simulink model "UberSpurs"  (R2015b)
settings: Solver=VariableStepAuto  StartTime=0.0  StopTime=5000  RelTol=1e-3
libraries: simulink x54
(part 1 of 6)
settings Model: Creator=tsprock3  LastModifiedBy=tsprock3
settings DebuggingCC: UnconnectedOutputMsg=error

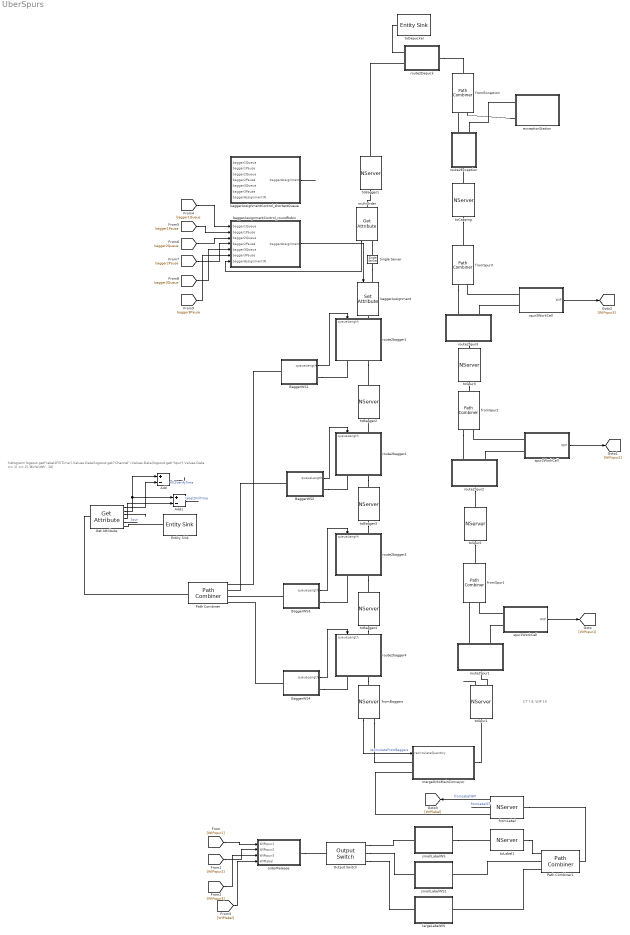
== system UberSpurs ==
  note: histogram(logsout.get('label2FillTime').Values.Data(logsout.get('Channel').Values.Data(logsout.get('Spur').Values.Data == 1) == 2),'BinWidth', 10)
  note: CT 7.8, WIP 19
  Add : Sum  Inputs=+-
  Add1 : Sum  Inputs=+-
  BaggerWS1 : Subsystem
  BaggerWS2 : Subsystem
  BaggerWS3 : Subsystem
  BaggerWS4 : Subsystem
  Entity Sink : EntitySink
  Get Attribute : GetAttribute  AttributeName=FillTime|VerifyTime|Channel|LabelTime|Spur  AttributeMissing=Error|Error|Error|Error|Error  AttributeDefaultValue=1|1|1|1|1  AttributeTreatAsVector=1|1|1|1|1  AttributeSendTiming=After entity departure|After entity departure|After entity departure|After entity departure|After entity departure  EvaluatedDefaultAttributeValue={ [];[];[];[];[]}
      settings: OutputPortMap=o1,o2,o3,o4,o5
  Output Switch : OutputSwitch  SwitchingCriterion=From attribute  AttributeName=Labeler  InitialConditionsOpt=on
  Path Combiner : PathCombiner  NumberInputPorts=4
  Path Combiner1 : PathCombiner
  Single Server : SingleServer  ServiceTime=0
  baggerAssignment : SetAttribute  AttributeName=Bagger  AttributeFrom=Signal port  EvaluatedAttributeValue={ []}
  baggerAssignmentControl_roundRobin : Stateflow chart  TreatAsAtomicUnit=on
  baggerAssignmentControl_shortestQueue : Stateflow chart  TreatAsAtomicUnit=on
  exceptionStation : Subsystem
  fromBaggers : NServer  NumberOfServers=12  ServiceTime=4.9  StatNumberInBlock=on
      settings: OutputPortMap=o1
  fromException : PathCombiner  NumberInputPorts=2
  fromLabel : NServer  NumberOfServers=45  ServiceTime=37  StatNumberInBlock=on  StatAverageWait=on
      settings: OutputPortMap=o1,o4
  fromSpur1 : PathCombiner  NumberInputPorts=2  InputPortPrecedence=Round robin
  fromSpur2 : PathCombiner  NumberInputPorts=2  InputPortPrecedence=Round robin
  fromSpur3 : PathCombiner  NumberInputPorts=2  InputPortPrecedence=Round robin
  largeLabelWS : Subsystem
  mergeOntoMainConveyor : Subsystem
  multiOrder : GetAttribute  AttributeName=Bagger  EvaluatedDefaultAttributeValue={ []}
      settings: OutputPortMap=o1
  orderRelease : Subsystem
  route2Depuck : Subsystem
  route2Exception : Subsystem
  route2Spur1 : Subsystem
  route2Spur2 : Subsystem
  route2Spur3 : Subsystem
  route2bagger1 : Subsystem
  route2bagger2 : Subsystem
  route2bagger3 : Subsystem
  route2bagger4 : Subsystem
  smallLabelWS : Subsystem
  smallLabelWS1 : Subsystem
  spur1WorkCell : Subsystem
  spur2WorkCell : Subsystem
  spur3WorkCell : Subsystem
  toBagger{1..4} (4 alike) : NServer  NumberOfServers=30  ServiceTime=12.1
  toCapping : NServer  NumberOfServers=25  ServiceTime=10.4
  toDepucker : EntitySink
  toLabel1 : NServer  NumberOfServers=22  ServiceTime=8
  toSpur1 : NServer  NumberOfServers=19  ServiceTime=7.79  StatNumberInBlock=on
      settings: OutputPortMap=o1
  toSpur2 : NServer  NumberOfServers=20  ServiceTime=8.3
  toSpur3 : NServer  NumberOfServers=20  ServiceTime=8.3
  wires:
  Add/1 -> ?  "fill2VerifyTime"
  Get Attribute/3 -> ?
  Get Attribute/2 -> Add1/1, Add/1
  Get Attribute/1 -> Add/2
  Add1/1 -> ?  "label2FillTime"
  Get Attribute/4 -> Add1/2
  spur1WorkCell/1(WIP) -> [WIPspur1]
  [WIPspur1] -> orderRelease/1(WIPspur1)
  BaggerWS4/1(queueLength) -> route2bagger4/1(queueLength)
  BaggerWS3/1(queueLength) -> route2bagger3/1(queueLength)
  BaggerWS2/1(queueLength) -> route2bagger2/1(queueLength)
  BaggerWS1/1(queueLength) -> route2bagger1/1(queueLength)
  spur2WorkCell/1(WIP) -> [WIPspur2]
  [WIPspur2] -> orderRelease/2(WIPspur2)
  fromLabel/2 -> ?  "fromLabelCT"
  fromLabel/1 -> [WIPlabel]  "fromLabelWIP"
  [WIPspur3] -> orderRelease/3(WIPspur3)
  [WIPlabel] -> orderRelease/4(WIPlabel)
  toSpur1/1 -> ?
  Get Attribute/5 -> ?  "Spur"
  spur3WorkCell/1(WIP) -> [WIPspur3]
  fromBaggers/1 -> mergeOntoMainConveyor/1(recirculateQuantity)  "recirculateFromBaggers"
  baggerAssignmentControl_roundRobin/1(baggerAssignment) -> baggerAssignment/1
  multiOrder/1 -> baggerAssignmentControl_roundRobin/7(baggerAssignmentIN)
  [bagger1Queue] -> baggerAssignmentControl_roundRobin/1(bagger1Queue)
  [bagger1Pause] -> baggerAssignmentControl_roundRobin/2(bagger1Pause)
  [bagger2Queue] -> baggerAssignmentControl_roundRobin/3(bagger2Queue)
  [bagger2Pause] -> baggerAssignmentControl_roundRobin/4(bagger2Pause)
  [bagger3Queue] -> baggerAssignmentControl_roundRobin/5(bagger3Queue)
  [bagger3Pause] -> baggerAssignmentControl_roundRobin/6(bagger3Pause)
  baggerAssignmentControl_shortestQueue/1(baggerAssignment) -> ?
  connections:
  Get Attribute/RConn1 -- Entity Sink/LConn1
  spur1WorkCell/LConn1 -- fromSpur1/LConn2
  toSpur1/RConn1 -- route2Spur1/LConn1
  route2Spur1/RConn2 -- spur1WorkCell/LConn2
  route2Spur1/RConn1 -- fromSpur1/LConn1
  BaggerWS1/LConn1 -- Path Combiner/LConn1
  BaggerWS3/LConn1 -- Path Combiner/LConn3
  Path Combiner/RConn1 -- Get Attribute/LConn1
  Output Switch/RConn2 -- smallLabelWS1/LConn1
  toLabel1/RConn1 -- Path Combiner1/LConn1
  BaggerWS4/RConn1 -- route2bagger4/RConn1
  route2bagger4/RConn2 -- fromBaggers/LConn1
  toBagger4/RConn1 -- route2bagger4/LConn1
  orderRelease/RConn1 -- Output Switch/LConn1
  BaggerWS3/RConn1 -- route2bagger3/RConn1
  route2bagger3/RConn2 -- toBagger4/LConn1
  BaggerWS2/LConn1 -- Path Combiner/LConn2
  toBagger3/RConn1 -- route2bagger3/LConn1
  route2bagger2/RConn2 -- toBagger3/LConn1
  BaggerWS2/RConn1 -- route2bagger2/RConn1
  toBagger2/RConn1 -- route2bagger2/LConn1
  route2bagger1/RConn2 -- toBagger2/LConn1
  BaggerWS1/RConn1 -- route2bagger1/RConn1
  toSpur2/LConn1 -- fromSpur1/RConn1
  Path Combiner1/LConn2 -- smallLabelWS1/RConn1
  fromLabel/LConn1 -- Path Combiner1/RConn1
  BaggerWS4/LConn1 -- Path Combiner/LConn4
  spur2WorkCell/LConn2 -- route2Spur2/RConn2
  route2Spur2/LConn1 -- toSpur2/RConn1
  fromSpur2/LConn1 -- route2Spur2/RConn1
  toSpur3/LConn1 -- fromSpur2/RConn1
  spur2WorkCell/LConn1 -- fromSpur2/LConn2
  spur3WorkCell/LConn1 -- fromSpur3/LConn2
  fromSpur3/LConn1 -- route2Spur3/RConn1
  spur3WorkCell/LConn2 -- route2Spur3/RConn2
  route2Spur3/LConn1 -- toSpur3/RConn1
  toCapping/LConn1 -- fromSpur3/RConn1
  toCapping/RConn1 -- route2Exception/LConn1
  route2Exception/RConn1 -- fromException/LConn1
  route2Exception/RConn2 -- exceptionStation/LConn1
  exceptionStation/LConn2 -- fromException/LConn2
  route2Depuck/LConn1 -- fromException/RConn1
  route2Depuck/RConn2 -- toBagger1/LConn1
  toDepucker/LConn1 -- route2Depuck/RConn1
  Path Combiner1/LConn3 -- largeLabelWS/RConn1
  Output Switch/RConn3 -- largeLabelWS/LConn1
  smallLabelWS/RConn1 -- toLabel1/LConn1
  Output Switch/RConn1 -- smallLabelWS/LConn1
  fromBaggers/RConn1 -- mergeOntoMainConveyor/LConn1
  mergeOntoMainConveyor/RConn1 -- toSpur1/LConn1
  fromLabel/RConn1 -- mergeOntoMainConveyor/LConn2
  baggerAssignment/RConn1 -- route2bagger1/LConn1
  multiOrder/LConn1 -- toBagger1/RConn1
  Single Server/RConn1 -- baggerAssignment/LConn1
  Single Server/LConn1 -- multiOrder/RConn1

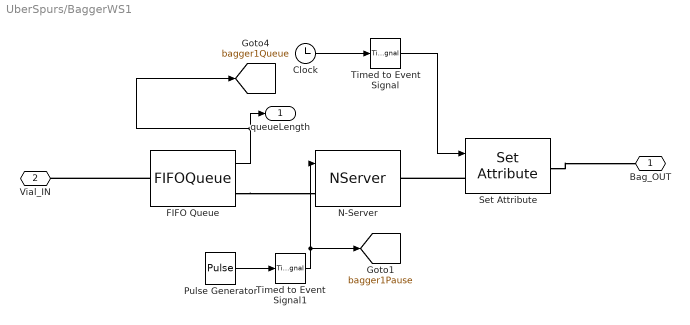
== system UberSpurs/BaggerWS1 ==
  Clock : Clock
  FIFO Queue : FIFOQueue  Capacity=26  StatNumberInBlock=on
      settings: OutputPortMap=o1
  N-Server : NServer  NumberOfServers=1  ServiceTime=6  AllowServiceControl=on
      settings: InputPortMap=u1
  Pulse Generator : DiscretePulseGenerator  PulseType=Time based  Period=100  PulseWidth=10
  Set Attribute : SetAttribute  AttributeName=BagTime  AttributeFrom=Signal port  EvaluatedAttributeValue={ []}
  Timed to Event Signal : TimedToEventSignal
  Timed to Event Signal1 : TimedToEventSignal
  Bag_OUT : PMIOPort  Port=1  Side=Left
  Vial_IN : PMIOPort  Port=2  Side=Right
  queueLength : Outport
  tag scope: bagger1Pause=global, bagger1Queue=global
  wires:
  Clock/1 -> Timed to Event Signal/1
  Timed to Event Signal/1 -> Set Attribute/1
  FIFO Queue/1 -> [bagger1Queue], queueLength/1
  Pulse Generator/1 -> Timed to Event Signal1/1
  Timed to Event Signal1/1 -> [bagger1Pause], N-Server/1
  connections:
  FIFO Queue/LConn1 -- Vial_IN/RConn1
  FIFO Queue/RConn1 -- N-Server/LConn1
  Set Attribute/LConn1 -- N-Server/RConn1
  Set Attribute/RConn1 -- Bag_OUT/RConn1

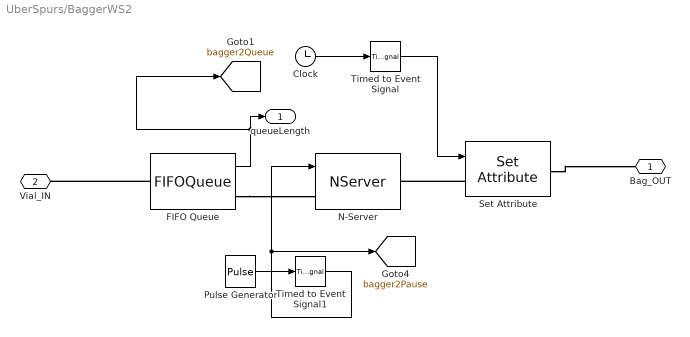
== system UberSpurs/BaggerWS2 ==
  Clock : Clock
  FIFO Queue : FIFOQueue  Capacity=26  StatNumberInBlock=on
      settings: OutputPortMap=o1
  N-Server : NServer  NumberOfServers=1  ServiceTime=6  AllowServiceControl=on
      settings: InputPortMap=u1
  Pulse Generator : DiscretePulseGenerator  PulseType=Time based  Period=100  PulseWidth=10  PhaseDelay=250
  Set Attribute : SetAttribute  AttributeName=BagTime  AttributeFrom=Signal port  EvaluatedAttributeValue={ []}
  Timed to Event Signal : TimedToEventSignal
  Timed to Event Signal1 : TimedToEventSignal
  Bag_OUT : PMIOPort  Port=1  Side=Left
  Vial_IN : PMIOPort  Port=2  Side=Right
  queueLength : Outport
  tag scope: bagger2Pause=global, bagger2Queue=global
  wires:
  Clock/1 -> Timed to Event Signal/1
  Timed to Event Signal/1 -> Set Attribute/1
  FIFO Queue/1 -> [bagger2Queue], queueLength/1
  Pulse Generator/1 -> Timed to Event Signal1/1
  Timed to Event Signal1/1 -> [bagger2Pause], N-Server/1
  connections:
  FIFO Queue/LConn1 -- Vial_IN/RConn1
  FIFO Queue/RConn1 -- N-Server/LConn1
  Set Attribute/LConn1 -- N-Server/RConn1
  Set Attribute/RConn1 -- Bag_OUT/RConn1

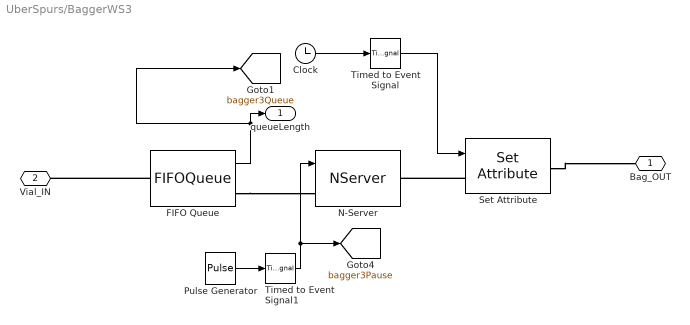
== system UberSpurs/BaggerWS3 ==
  Clock : Clock
  FIFO Queue : FIFOQueue  Capacity=26  StatNumberInBlock=on
      settings: OutputPortMap=o1
  N-Server : NServer  NumberOfServers=1  ServiceTime=6  AllowServiceControl=on
      settings: InputPortMap=u1
  Pulse Generator : DiscretePulseGenerator  PulseType=Time based  Period=100  PulseWidth=10  PhaseDelay=500
  Set Attribute : SetAttribute  AttributeName=BagTime  AttributeFrom=Signal port  EvaluatedAttributeValue={ []}
  Timed to Event Signal : TimedToEventSignal
  Timed to Event Signal1 : TimedToEventSignal
  Bag_OUT : PMIOPort  Port=1  Side=Left
  Vial_IN : PMIOPort  Port=2  Side=Right
  queueLength : Outport
  tag scope: bagger3Pause=global, bagger3Queue=global
  wires:
  Clock/1 -> Timed to Event Signal/1
  Timed to Event Signal/1 -> Set Attribute/1
  FIFO Queue/1 -> [bagger3Queue], queueLength/1
  Pulse Generator/1 -> Timed to Event Signal1/1
  Timed to Event Signal1/1 -> [bagger3Pause], N-Server/1
  connections:
  FIFO Queue/LConn1 -- Vial_IN/RConn1
  FIFO Queue/RConn1 -- N-Server/LConn1
  Set Attribute/LConn1 -- N-Server/RConn1
  Set Attribute/RConn1 -- Bag_OUT/RConn1

== system UberSpurs/BaggerWS4 ==
  Clock : Clock
  FIFO Queue : FIFOQueue  Capacity=26  StatNumberInBlock=on
      settings: OutputPortMap=o1
  N-Server : NServer  NumberOfServers=1  ServiceTime=6  AllowServiceControl=on
      settings: InputPortMap=u1
  Pulse Generator : DiscretePulseGenerator  PulseType=Time based  Period=100  PulseWidth=10  PhaseDelay=750
  Set Attribute : SetAttribute  AttributeName=BagTime  AttributeFrom=Signal port  EvaluatedAttributeValue={ []}
  Timed to Event Signal : TimedToEventSignal
  Timed to Event Signal1 : TimedToEventSignal
  Bag_OUT : PMIOPort  Port=1  Side=Left
  Vial_IN : PMIOPort  Port=2  Side=Right
  queueLength : Outport
  wires:
  Clock/1 -> Timed to Event Signal/1
  Timed to Event Signal/1 -> Set Attribute/1
  FIFO Queue/1 -> queueLength/1
  Pulse Generator/1 -> Timed to Event Signal1/1
  Timed to Event Signal1/1 -> N-Server/1
  connections:
  FIFO Queue/LConn1 -- Vial_IN/RConn1
  FIFO Queue/RConn1 -- N-Server/LConn1
  Set Attribute/LConn1 -- N-Server/RConn1
  Set Attribute/RConn1 -- Bag_OUT/RConn1

== system UberSpurs/exceptionStation ==
  Clock : Clock
  Event-Based Random Number : EventBasedRandomNumber  Distribution=Gaussian (normal)  meanNorm=120  stdNorm=30  Seed=15123
  FIFO Queue : FIFOQueue  Capacity=100
  N-Server : NServer  NumberOfServers=inf  ServiceTimeFrom=Signal port t
  Set Attribute1 : SetAttribute  AttributeName=VerifyTime  AttributeFrom=Signal port  EvaluatedAttributeValue={ []}
  Timed to Event Signal : TimedToEventSignal
  fromCap : PMIOPort  Port=1  Side=Left
  toBagger : PMIOPort  Port=2  Side=Left
  wires:
  Event-Based Random Number/1 -> N-Server/1
  Clock/1 -> Timed to Event Signal/1
  Timed to Event Signal/1 -> Set Attribute1/1
  connections:
  N-Server/LConn1 -- FIFO Queue/RConn1
  N-Server/RConn1 -- Set Attribute1/LConn1
  fromCap/RConn1 -- FIFO Queue/LConn1
  toBagger/RConn1 -- Set Attribute1/RConn1

== system UberSpurs/largeLabelWS ==
  Queue : FIFOQueue
  Server : NServer  NumberOfServers=1  ServiceTime=3.5
  vialOUT : PMIOPort  Port=1  Side=Right
  vialIn : PMIOPort  Port=2  Side=Left
  connections:
  vialIn/RConn1 -- Queue/LConn1
  Server/LConn1 -- Queue/RConn1
  Server/RConn1 -- vialOUT/RConn1

== system UberSpurs/mergeOntoMainConveyor ==
  recirculateQuantity : Inport
  Path Combiner2 : PathCombiner  NumberInputPorts=2  InputPortPrecedence=Round robin
  Single Server : SingleServer  ServiceTime=0
  fromMerge : NServer  NumberOfServers=1  ServiceTime=.4
  mergeControl : Stateflow chart  TreatAsAtomicUnit=on
  toMerge : NServer  NumberOfServers=1  ServiceTime=.4  AllowServiceControl=on  BlockWhileSignalOn=on
      settings: InputPortMap=u1
  toMerge1 : NServer  NumberOfServers=1  ServiceTime=.2  AllowServiceControl=on  BlockWhileSignalOn=on
      settings: InputPortMap=u1
  fromRecirculate : PMIOPort  Port=1  Side=Left
  toUberSpurs : PMIOPort  Port=2  Side=Right
  fromLabel : PMIOPort  Port=3  Side=Left
  wires:
  recirculateQuantity/1 -> mergeControl/1(recirculateQueue)
  mergeControl/1(merge) -> toMerge1/1
  mergeControl/2(recirculate) -> toMerge/1
  connections:
  fromLabel/RConn1 -- toMerge1/LConn1
  fromMerge/RConn1 -- toUberSpurs/RConn1
  Single Server/RConn1 -- toMerge/LConn1
  Path Combiner2/RConn1 -- fromMerge/LConn1
  fromRecirculate/RConn1 -- Single Server/LConn1
  toMerge/RConn1 -- Path Combiner2/LConn1
  toMerge1/RConn1 -- Path Combiner2/LConn2

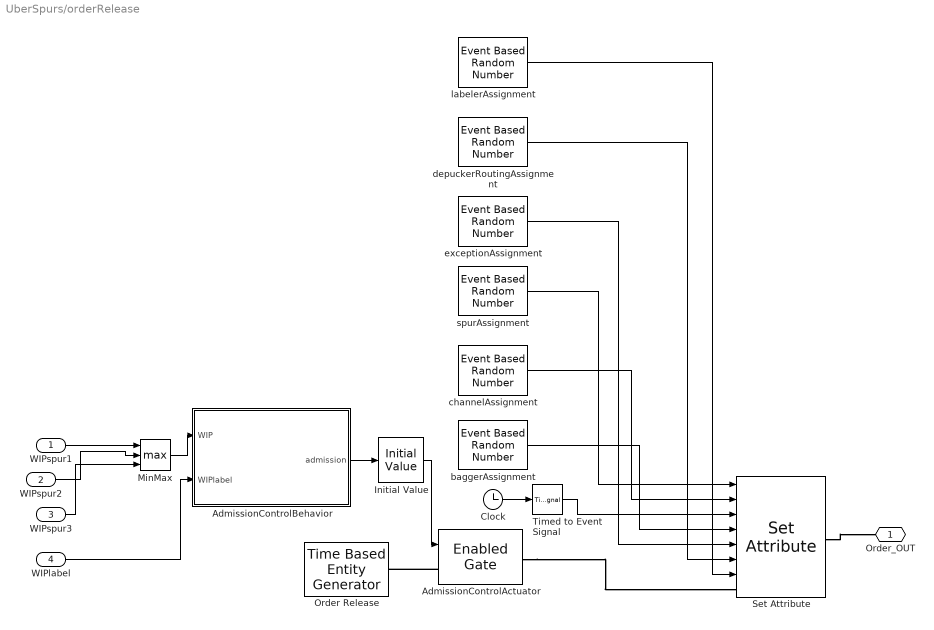
== system UberSpurs/orderRelease ==
  WIPspur1 : Inport
  WIPspur2 : Inport  Port=2
  WIPspur3 : Inport  Port=3
  WIPlabel : Inport  Port=4
  AdmissionControlActuator : EnabledGate
  AdmissionControlBehavior : Stateflow chart  TreatAsAtomicUnit=on
  Clock : Clock
  Initial Value : InitialValue
  MinMax : MinMax  Function=max  Inputs=3
  Order Release : TimeBasedEntityGenerator  Period=.78  InitialSeed=16773
  Set Attribute : SetAttribute  AttributeName=Spur|Channel|LabelTime|FillTime|VerifyTime|BagTime|Bagger|Exception|Depucker|Labeler  AttributeFrom=Signal port|Signal port|Signal port|Dialog|Dialog|Dialog|Signal port|Signal port|Signal port|Signal port  AttributeValue=1|1|1|0|0|0|1|1|1|1  AttributeTreatAsVector=1|1|1|1|1|1|1|1|1|1  EvaluatedAttributeValue={ [];[];[];0;0;0;[];[];[];[]}
      settings: InputPortMap=u0,u1,u2,u6,u7,u8,u9
  Timed to Event Signal : TimedToEventSignal
  baggerAssignment : EventBasedRandomNumber  Distribution=Arbitrary discrete  valueVecDisc=[1 2 3 4]  probVecDisc=[0.30 0.30 0.30 0.10]  Seed=18340
  channelAssignment : EventBasedRandomNumber  Distribution=Arbitrary discrete  valueVecDisc=[1 2 3 4 5 6 7 8 9 10 11 12 13 14 15 16 17 18]  probVecDisc=[0.065 0.055 0.055 0.055 0.055 0.055 0.055 0.055 0.055 0.055 0.055 0.055 0.055 0.055 0.055 0.055 0.055 0.055]  Seed=21557
  depuckerRoutingAssignment : EventBasedRandomNumber  Distribution=Arbitrary discrete  valueVecDisc=[1 2]  probVecDisc=[0.23 0.77]  Seed=62554
  exceptionAssignment : EventBasedRandomNumber  Distribution=Arbitrary discrete  probVecDisc=[0.927 0.073]  Seed=235
  labelerAssignment : EventBasedRandomNumber  Distribution=Arbitrary discrete  valueVecDisc=[1 2 3]  probVecDisc=[0.4 0.4 0.2]
  spurAssignment : EventBasedRandomNumber  Distribution=Arbitrary discrete  valueVecDisc=[1 2 3]  probVecDisc=[0.33 0.33 0.34]  Seed=27991
  Order_OUT : PMIOPort  Port=1  Side=Right
  wires:
  Clock/1 -> Timed to Event Signal/1
  Timed to Event Signal/1 -> Set Attribute/3
  channelAssignment/1 -> Set Attribute/2
  MinMax/1 -> AdmissionControlBehavior/1(WIP)
  WIPspur2/1 -> MinMax/2
  baggerAssignment/1 -> Set Attribute/4
  WIPspur1/1 -> MinMax/1
  WIPspur3/1 -> MinMax/3
  WIPlabel/1 -> AdmissionControlBehavior/2(WIPlabel)
  AdmissionControlBehavior/1(admission) -> Initial Value/1
  Initial Value/1 -> AdmissionControlActuator/1
  exceptionAssignment/1 -> Set Attribute/5
  spurAssignment/1 -> Set Attribute/1
  depuckerRoutingAssignment/1 -> Set Attribute/6
  labelerAssignment/1 -> Set Attribute/7
  connections:
  AdmissionControlActuator/LConn1 -- Order Release/RConn1
  AdmissionControlActuator/RConn1 -- Set Attribute/LConn1
  Set Attribute/RConn1 -- Order_OUT/RConn1

== system UberSpurs/route2Depuck ==
  Output Switch : OutputSwitch  NumberOutputPorts=2  SwitchingCriterion=From attribute  AttributeName=Depucker  InitialConditionsOpt=on
  Single Server : SingleServer  ServiceTime=0
  toDepucker : PMIOPort  Port=1  Side=Right
  toBagger : PMIOPort  Port=2  Side=Right
  fromCap : PMIOPort  Port=3  Side=Left
  connections:
  Single Server/RConn1 -- Output Switch/LConn1
  Output Switch/RConn1 -- toDepucker/RConn1
  Output Switch/RConn2 -- toBagger/RConn1
  fromCap/RConn1 -- Single Server/LConn1

== system UberSpurs/route2Exception ==
  Get Attribute1 : GetAttribute  AttributeName=Exception  EvaluatedDefaultAttributeValue={ []}
      settings: OutputPortMap=o1
  Output Switch : OutputSwitch  NumberOutputPorts=2  SwitchingCriterion=From signal port p  InitialConditionsOpt=on
  Single Server : SingleServer  ServiceTime=0
  exceptions : Stateflow chart  TreatAsAtomicUnit=on
  toBagger : PMIOPort  Port=1  Side=Right
  toExceptions : PMIOPort  Port=2  Side=Right
  fromCap : PMIOPort  Port=3  Side=Left
  wires:
  Get Attribute1/1 -> exceptions/1(exceptions)
  exceptions/1(route) -> Output Switch/1
  connections:
  Get Attribute1/LConn1 -- fromCap/RConn1
  Get Attribute1/RConn1 -- Single Server/LConn1
  Single Server/RConn1 -- Output Switch/LConn1
  Output Switch/RConn1 -- toBagger/RConn1
  Output Switch/RConn2 -- toExceptions/RConn1

== system UberSpurs/route2Spur1 ==
  Get Attribute1 : GetAttribute  AttributeName=Spur|VerifyTime  AttributeMissing=Error|Error  AttributeDefaultValue=1|1  AttributeTreatAsVector=1|1  AttributeSendTiming=After entity departure|After entity departure  EvaluatedDefaultAttributeValue={ [];[]}
      settings: OutputPortMap=o1,o2
  Single Server : SingleServer  ServiceTime=0
  offSpur1 : OutputSwitch  NumberOutputPorts=2  SwitchingCriterion=From signal port p  InitialConditionsOpt=on
  routingControl : Stateflow chart  TreatAsAtomicUnit=on
  toMHS : PMIOPort  Port=1  Side=Right
  toSpur : PMIOPort  Port=2  Side=Right
  fromMHS : PMIOPort  Port=3  Side=Left
  wires:
  Get Attribute1/1 -> routingControl/1(entitySpur)
  routingControl/1(route) -> offSpur1/1
  Get Attribute1/2 -> routingControl/2(VerifyTime)
  connections:
  offSpur1/RConn2 -- toSpur/RConn1
  fromMHS/RConn1 -- Get Attribute1/LConn1
  offSpur1/RConn1 -- toMHS/RConn1
  Single Server/LConn1 -- Get Attribute1/RConn1
  Single Server/RConn1 -- offSpur1/LConn1

== system UberSpurs/route2Spur2 ==
  Get Attribute1 : GetAttribute  AttributeName=Spur|VerifyTime  AttributeMissing=Error|Error  AttributeDefaultValue=1|1  AttributeTreatAsVector=1|1  AttributeSendTiming=After entity departure|After entity departure  EvaluatedDefaultAttributeValue={ [];[]}
      settings: OutputPortMap=o1,o2
  Single Server : SingleServer  ServiceTime=0
  offSpur1 : OutputSwitch  NumberOutputPorts=2  SwitchingCriterion=From signal port p  InitialConditionsOpt=on
  routingControl : Stateflow chart  TreatAsAtomicUnit=on
  toMHS : PMIOPort  Port=1  Side=Right
  toSpur : PMIOPort  Port=2  Side=Right
  fromMHS : PMIOPort  Port=3  Side=Left
  wires:
  Get Attribute1/1 -> routingControl/1(entitySpur)
  routingControl/1(route) -> offSpur1/1
  Get Attribute1/2 -> routingControl/2(VerifyTime)
  connections:
  offSpur1/RConn2 -- toSpur/RConn1
  fromMHS/RConn1 -- Get Attribute1/LConn1
  offSpur1/RConn1 -- toMHS/RConn1
  Single Server/LConn1 -- Get Attribute1/RConn1
  Single Server/RConn1 -- offSpur1/LConn1

== system UberSpurs/route2Spur3 ==
  Get Attribute1 : GetAttribute  AttributeName=Spur|VerifyTime  AttributeMissing=Error|Error  AttributeDefaultValue=1|1  AttributeTreatAsVector=1|1  AttributeSendTiming=After entity departure|After entity departure  EvaluatedDefaultAttributeValue={ [];[]}
      settings: OutputPortMap=o1,o2
  Single Server : SingleServer  ServiceTime=0
  offSpur1 : OutputSwitch  NumberOutputPorts=2  SwitchingCriterion=From signal port p  InitialConditionsOpt=on
  routingControl : Stateflow chart  TreatAsAtomicUnit=on
  toMHS : PMIOPort  Port=1  Side=Right
  toSpur : PMIOPort  Port=2  Side=Right
  fromMHS : PMIOPort  Port=3  Side=Left
  wires:
  Get Attribute1/1 -> routingControl/1(entitySpur)
  routingControl/1(route) -> offSpur1/1
  Get Attribute1/2 -> routingControl/2(VerifyTime)
  connections:
  offSpur1/RConn2 -- toSpur/RConn1
  fromMHS/RConn1 -- Get Attribute1/LConn1
  offSpur1/RConn1 -- toMHS/RConn1
  Single Server/LConn1 -- Get Attribute1/RConn1
  Single Server/RConn1 -- offSpur1/LConn1

== system UberSpurs/route2bagger1 ==
  queueLength : Inport
  Get Attribute1 : GetAttribute  AttributeName=Bagger  EvaluatedDefaultAttributeValue={ []}
      settings: OutputPortMap=o1
  Single Server : SingleServer  ServiceTime=0
  offBagger : OutputSwitch  NumberOutputPorts=2  SwitchingCriterion=From signal port p  InitialConditionsOpt=on
  routingControl : Stateflow chart  TreatAsAtomicUnit=on
  toBagger : PMIOPort  Port=1  Side=Right
  toMHS : PMIOPort  Port=2  Side=Right
  fromMHS : PMIOPort  Port=3  Side=Left
  wires:
  Get Attribute1/1 -> routingControl/1(entityBagger)
  routingControl/1(route) -> offBagger/1
  queueLength/1 -> routingControl/2(queueLength)
  connections:
  offBagger/RConn2 -- toBagger/RConn1
  fromMHS/RConn1 -- Get Attribute1/LConn1
  offBagger/RConn1 -- toMHS/RConn1
  Single Server/LConn1 -- Get Attribute1/RConn1
  Single Server/RConn1 -- offBagger/LConn1

== system UberSpurs/route2bagger2 ==
  queueLength : Inport
  Get Attribute1 : GetAttribute  AttributeName=Bagger  EvaluatedDefaultAttributeValue={ []}
      settings: OutputPortMap=o1
  Single Server : SingleServer  ServiceTime=0
  offBagger : OutputSwitch  NumberOutputPorts=2  SwitchingCriterion=From signal port p  InitialConditionsOpt=on
  routingControl : Stateflow chart  TreatAsAtomicUnit=on
  toBagger : PMIOPort  Port=1  Side=Right
  toMHS : PMIOPort  Port=2  Side=Right
  fromMHS : PMIOPort  Port=3  Side=Left
  wires:
  Get Attribute1/1 -> routingControl/1(entityBagger)
  routingControl/1(route) -> offBagger/1
  queueLength/1 -> routingControl/2(queueLength)
  connections:
  offBagger/RConn2 -- toBagger/RConn1
  fromMHS/RConn1 -- Get Attribute1/LConn1
  offBagger/RConn1 -- toMHS/RConn1
  Single Server/LConn1 -- Get Attribute1/RConn1
  Single Server/RConn1 -- offBagger/LConn1

== system UberSpurs/route2bagger3 ==
  queueLength : Inport
  Get Attribute1 : GetAttribute  AttributeName=Bagger  EvaluatedDefaultAttributeValue={ []}
      settings: OutputPortMap=o1
  Single Server : SingleServer  ServiceTime=0
  offBagger : OutputSwitch  NumberOutputPorts=2  SwitchingCriterion=From signal port p  InitialConditionsOpt=on
  routingControl : Stateflow chart  TreatAsAtomicUnit=on
  toBagger : PMIOPort  Port=1  Side=Right
  toMHS : PMIOPort  Port=2  Side=Right
  fromMHS : PMIOPort  Port=3  Side=Left
  wires:
  Get Attribute1/1 -> routingControl/1(entityBagger)
  routingControl/1(route) -> offBagger/1
  queueLength/1 -> routingControl/2(queueLength)
  connections:
  offBagger/RConn2 -- toBagger/RConn1
  fromMHS/RConn1 -- Get Attribute1/LConn1
  offBagger/RConn1 -- toMHS/RConn1
  Single Server/LConn1 -- Get Attribute1/RConn1
  Single Server/RConn1 -- offBagger/LConn1

== system UberSpurs/route2bagger4 ==
  queueLength : Inport
  Get Attribute1 : GetAttribute  AttributeName=Bagger  EvaluatedDefaultAttributeValue={ []}
      settings: OutputPortMap=o1
  Single Server : SingleServer  ServiceTime=0
  offBagger : OutputSwitch  NumberOutputPorts=2  SwitchingCriterion=From signal port p  InitialConditionsOpt=on
  routingControl : Stateflow chart  TreatAsAtomicUnit=on
  toBagger : PMIOPort  Port=1  Side=Right
  toMHS : PMIOPort  Port=2  Side=Right
  fromMHS : PMIOPort  Port=3  Side=Left
  wires:
  Get Attribute1/1 -> routingControl/1(entityBagger)
  routingControl/1(route) -> offBagger/1
  queueLength/1 -> routingControl/2(queueLength)
  connections:
  offBagger/RConn2 -- toBagger/RConn1
  fromMHS/RConn1 -- Get Attribute1/LConn1
  offBagger/RConn1 -- toMHS/RConn1
  Single Server/LConn1 -- Get Attribute1/RConn1
  Single Server/RConn1 -- offBagger/LConn1

== system UberSpurs/smallLabelWS ==
  Queue : FIFOQueue
  Server : NServer  NumberOfServers=1  ServiceTime=3.5
  vialOUT : PMIOPort  Port=1  Side=Right
  vialIn : PMIOPort  Port=2  Side=Left
  connections:
  vialIn/RConn1 -- Queue/LConn1
  Server/LConn1 -- Queue/RConn1
  Server/RConn1 -- vialOUT/RConn1

== system UberSpurs/smallLabelWS1 ==
  Queue : FIFOQueue
  Server : NServer  NumberOfServers=1  ServiceTime=3.5
  vialOUT : PMIOPort  Port=1  Side=Right
  vialIn : PMIOPort  Port=2  Side=Left
  connections:
  vialIn/RConn1 -- Queue/LConn1
  Server/LConn1 -- Queue/RConn1
  Server/RConn1 -- vialOUT/RConn1

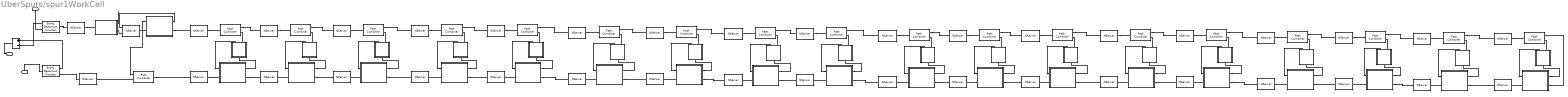
== system UberSpurs/spur1WorkCell ==
  Add1 : Sum  Inputs=+-
  INFlowCount : EntityDepartureCounter  NumberDepartedToSignal=on  NumberDepartedToAttribute=off
  OUTFlowCount : EntityDepartureCounter  NumberDepartedToSignal=on  NumberDepartedToAttribute=off
  combineRecirculate : PathCombiner  NumberInputPorts=2
  fillChannel1 : Subsystem
  fillChannel10 : Subsystem
  fillChannel11 : Subsystem
  fillChannel12 : Subsystem
  fillChannel13 : Subsystem
  fillChannel14 : Subsystem
  fillChannel15 : Subsystem
  fillChannel16 : Subsystem
  fillChannel17 : Subsystem
  fillChannel18 : Subsystem
  fillChannel2 : Subsystem
  fillChannel3 : Subsystem
  fillChannel4 : Subsystem
  fillChannel5 : Subsystem
  fillChannel6 : Subsystem
  fillChannel7 : Subsystem
  fillChannel8 : Subsystem
  fillChannel9 : Subsystem
  fromChannel{1..18} (18 alike) : PathCombiner  NumberInputPorts=2  InputPortPrecedence=Round robin
  route2Channel1 : Subsystem
  route2Channel10 : Subsystem
  route2Channel11 : Subsystem
  route2Channel12 : Subsystem
  route2Channel13 : Subsystem
  route2Channel14 : Subsystem
  route2Channel15 : Subsystem
  route2Channel16 : Subsystem
  route2Channel17 : Subsystem
  route2Channel18 : Subsystem
  route2Channel2 : Subsystem
  route2Channel3 : Subsystem
  route2Channel4 : Subsystem
  route2Channel5 : Subsystem
  route2Channel6 : Subsystem
  route2Channel7 : Subsystem
  route2Channel8 : Subsystem
  route2Channel9 : Subsystem
  route2recirculate : Subsystem
  toChannel : NServer  NumberOfServers=15  ServiceTime=6
  toChannel{1..18} (18 alike) : NServer  NumberOfServers=2  ServiceTime=0.8
  toMainConveyor : NServer  ServiceTime=2
  toRecirculate : NServer  NumberOfServers=3
  toVerify : NServer  NumberOfServers=12  ServiceTime=5  StatNumberInBlock=on
      settings: OutputPortMap=o1
  toVerify{1..17} (17 alike) : NServer  NumberOfServers=2  ServiceTime=0.8
  verifyWorkstation : Subsystem
  toMHS : PMIOPort  Port=1  Side=Left
  fromMHS : PMIOPort  Port=2  Side=Left
  WIP : Outport
  wires:
  fillChannel1/1(serverAvailable) -> route2Channel1/1(serverAvailable)
  INFlowCount/1 -> Add1/1
  OUTFlowCount/1 -> Add1/2
  Add1/1 -> WIP/1
  fillChannel2/1(serverAvailable) -> route2Channel2/1(serverAvailable)
  fillChannel3/1(serverAvailable) -> route2Channel3/1(serverAvailable)
  fillChannel4/1(serverAvailable) -> route2Channel4/1(serverAvailable)
  fillChannel5/1(serverAvailable) -> route2Channel5/1(serverAvailable)
  fillChannel6/1(serverAvailable) -> route2Channel6/1(serverAvailable)
  fillChannel7/1(serverAvailable) -> route2Channel7/1(serverAvailable)
  fillChannel8/1(serverAvailable) -> route2Channel8/1(serverAvailable)
  fillChannel9/1(serverAvailable) -> route2Channel9/1(serverAvailable)
  fillChannel10/1(serverAvailable) -> route2Channel10/1(serverAvailable)
  fillChannel11/1(serverAvailable) -> route2Channel11/1(serverAvailable)
  fillChannel12/1(serverAvailable) -> route2Channel12/1(serverAvailable)
  fillChannel13/1(serverAvailable) -> route2Channel13/1(serverAvailable)
  fillChannel14/1(serverAvailable) -> route2Channel14/1(serverAvailable)
  fillChannel15/1(serverAvailable) -> route2Channel15/1(serverAvailable)
  fillChannel16/1(serverAvailable) -> route2Channel16/1(serverAvailable)
  fillChannel17/1(serverAvailable) -> route2Channel17/1(serverAvailable)
  fillChannel18/1(serverAvailable) -> route2Channel18/1(serverAvailable)
  toVerify/1 -> route2recirculate/1(verifyQueueLength)
  verifyWorkstation/1(queueLength) -> ?
  connections:
  fillChannel1/LConn1 -- route2Channel1/RConn1
  toChannel1/RConn1 -- route2Channel1/LConn1
  combineRecirculate/RConn1 -- toChannel1/LConn1
  route2recirculate/RConn1 -- combineRecirculate/LConn1
  OUTFlowCount/RConn1 -- toMHS/RConn1
  fromMHS/RConn1 -- INFlowCount/LConn1
  fillChannel1/RConn1 -- fromChannel1/LConn2
  toRecirculate/LConn1 -- fromChannel1/RConn1
  route2recirculate/LConn1 -- toRecirculate/RConn1
  route2Channel2/RConn1 -- fillChannel2/LConn1
  fillChannel2/RConn1 -- fromChannel2/LConn2
  route2Channel2/LConn1 -- toChannel2/RConn1
  toVerify1/LConn1 -- fromChannel2/RConn1
  route2Channel3/RConn1 -- fillChannel3/LConn1
  fillChannel3/RConn1 -- fromChannel3/LConn2
  route2Channel3/LConn1 -- toChannel3/RConn1
  toVerify2/LConn1 -- fromChannel3/RConn1
  route2Channel4/RConn1 -- fillChannel4/LConn1
  fillChannel4/RConn1 -- fromChannel4/LConn2
  route2Channel4/LConn1 -- toChannel4/RConn1
  toVerify3/LConn1 -- fromChannel4/RConn1
  route2Channel5/RConn1 -- fillChannel5/LConn1
  fillChannel5/RConn1 -- fromChannel5/LConn2
  route2Channel5/LConn1 -- toChannel5/RConn1
  toVerify4/LConn1 -- fromChannel5/RConn1
  route2Channel6/RConn1 -- fillChannel6/LConn1
  fillChannel6/RConn1 -- fromChannel6/LConn2
  route2Channel6/LConn1 -- toChannel6/RConn1
  toVerify5/LConn1 -- fromChannel6/RConn1
  route2Channel7/RConn1 -- fillChannel7/LConn1
  fillChannel7/RConn1 -- fromChannel7/LConn2
  route2Channel7/LConn1 -- toChannel7/RConn1
  toVerify6/LConn1 -- fromChannel7/RConn1
  route2Channel8/RConn1 -- fillChannel8/LConn1
  fillChannel8/RConn1 -- fromChannel8/LConn2
  route2Channel8/LConn1 -- toChannel8/RConn1
  toVerify7/LConn1 -- fromChannel8/RConn1
  route2Channel9/RConn1 -- fillChannel9/LConn1
  fillChannel9/RConn1 -- fromChannel9/LConn2
  route2Channel9/LConn1 -- toChannel9/RConn1
  toVerify8/LConn1 -- fromChannel9/RConn1
  fromChannel1/LConn1 -- toVerify1/RConn1
  route2Channel1/RConn2 -- toChannel2/LConn1
  route2Channel2/RConn2 -- toChannel3/LConn1
  fromChannel2/LConn1 -- toVerify2/RConn1
  fromChannel3/LConn1 -- toVerify3/RConn1
  route2Channel3/RConn2 -- toChannel4/LConn1
  fromChannel4/LConn1 -- toVerify4/RConn1
  route2Channel4/RConn2 -- toChannel5/LConn1
  fromChannel5/LConn1 -- toVerify5/RConn1
  route2Channel5/RConn2 -- toChannel6/LConn1
  fromChannel6/LConn1 -- toVerify6/RConn1
  route2Channel6/RConn2 -- toChannel7/LConn1
  fromChannel7/LConn1 -- toVerify7/RConn1
  route2Channel7/RConn2 -- toChannel8/LConn1
  fromChannel8/LConn1 -- toVerify8/RConn1
  route2Channel8/RConn2 -- toChannel9/LConn1
  route2Channel10/RConn2 -- toChannel11/LConn1
  route2Channel12/LConn1 -- toChannel12/RConn1
  route2Channel18/RConn1 -- fillChannel18/LConn1
  fromChannel17/LConn1 -- toVerify17/RConn1
  route2Channel13/RConn2 -- toChannel14/LConn1
  toVerify11/LConn1 -- fromChannel12/RConn1
  fillChannel10/RConn1 -- fromChannel10/LConn2
  fillChannel16/RConn1 -- fromChannel16/LConn2
  toVerify15/LConn1 -- fromChannel16/RConn1
  fromChannel14/LConn1 -- toVerify14/RConn1
  fillChannel15/RConn1 -- fromChannel15/LConn2
  toVerify14/LConn1 -- fromChannel15/RConn1
  route2Channel17/RConn2 -- toChannel18/LConn1
  fromChannel10/LConn1 -- toVerify10/RConn1
  toVerify17/LConn1 -- fromChannel18/RConn1
  route2Channel15/RConn2 -- toChannel16/LConn1
  route2Channel16/LConn1 -- toChannel16/RConn1
  route2Channel11/RConn2 -- toChannel12/LConn1
  toVerify9/LConn1 -- fromChannel10/RConn1
  route2Channel16/RConn2 -- toChannel17/LConn1
  fromChannel15/LConn1 -- toVerify15/RConn1
  toVerify12/LConn1 -- fromChannel13/RConn1
  route2Channel16/RConn1 -- fillChannel16/LConn1
  fromChannel13/LConn1 -- toVerify13/RConn1
  route2Channel15/RConn1 -- fillChannel15/LConn1
  fromChannel16/LConn1 -- toVerify16/RConn1
  route2Channel12/RConn1 -- fillChannel12/LConn1
  fillChannel18/RConn1 -- fromChannel18/LConn2
  route2Channel15/LConn1 -- toChannel15/RConn1
  route2Channel12/RConn2 -- toChannel13/LConn1
  route2Channel18/LConn1 -- toChannel18/RConn1
  fillChannel12/RConn1 -- fromChannel12/LConn2
  route2Channel14/RConn2 -- toChannel15/LConn1
  fromChannel11/LConn1 -- toVerify11/RConn1
  fromChannel12/LConn1 -- toVerify12/RConn1
  route2Channel13/LConn1 -- toChannel13/RConn1
  route2Channel10/LConn1 -- toChannel10/RConn1
  toVerify13/LConn1 -- fromChannel14/RConn1
  route2Channel17/RConn1 -- fillChannel17/LConn1
  fillChannel14/RConn1 -- fromChannel14/LConn2
  fillChannel11/RConn1 -- fromChannel11/LConn2
  route2Channel10/RConn1 -- fillChannel10/LConn1
  route2Channel11/LConn1 -- toChannel11/RConn1
  fillChannel17/RConn1 -- fromChannel17/LConn2
  route2Channel17/LConn1 -- toChannel17/RConn1
  route2Channel14/LConn1 -- toChannel14/RConn1
  toVerify16/LConn1 -- fromChannel17/RConn1
  route2Channel13/RConn1 -- fillChannel13/LConn1
  fillChannel13/RConn1 -- fromChannel13/LConn2
  route2Channel14/RConn1 -- fillChannel14/LConn1
  route2Channel11/RConn1 -- fillChannel11/LConn1
  toVerify10/LConn1 -- fromChannel11/RConn1
  fromChannel9/LConn1 -- toVerify9/RConn1
  route2Channel9/RConn2 -- toChannel10/LConn1
  route2Channel18/RConn2 -- fromChannel18/LConn1
  toChannel/RConn1 -- combineRecirculate/LConn2
  INFlowCount/RConn1 -- toChannel/LConn1
  toVerify/RConn1 -- verifyWorkstation/RConn1
  toVerify/LConn1 -- route2recirculate/RConn2
  OUTFlowCount/LConn1 -- toMainConveyor/RConn1
  toMainConveyor/LConn1 -- verifyWorkstation/LConn1

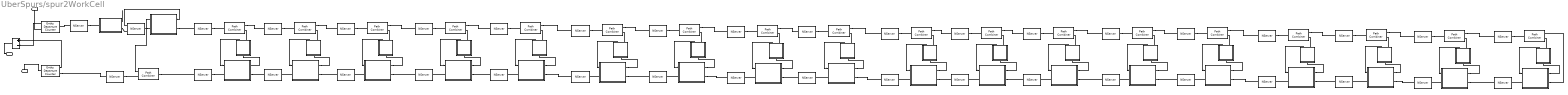
== system UberSpurs/spur2WorkCell ==
  Add1 : Sum  Inputs=+-
  INFlowCount : EntityDepartureCounter  NumberDepartedToSignal=on  NumberDepartedToAttribute=off
  OUTFlowCount : EntityDepartureCounter  NumberDepartedToSignal=on  NumberDepartedToAttribute=off
  combineRecirculate : PathCombiner  NumberInputPorts=2
  fillChannel1 : Subsystem
  fillChannel10 : Subsystem
  fillChannel11 : Subsystem
  fillChannel12 : Subsystem
  fillChannel13 : Subsystem
  fillChannel14 : Subsystem
  fillChannel15 : Subsystem
  fillChannel16 : Subsystem
  fillChannel17 : Subsystem
  fillChannel18 : Subsystem
  fillChannel2 : Subsystem
  fillChannel3 : Subsystem
  fillChannel4 : Subsystem
  fillChannel5 : Subsystem
  fillChannel6 : Subsystem
  fillChannel7 : Subsystem
  fillChannel8 : Subsystem
  fillChannel9 : Subsystem
  fromChannel{1..18} (18 alike) : PathCombiner  NumberInputPorts=2
  route2Channel1 : Subsystem
  route2Channel10 : Subsystem
  route2Channel11 : Subsystem
  route2Channel12 : Subsystem
  route2Channel13 : Subsystem
  route2Channel14 : Subsystem
  route2Channel15 : Subsystem
  route2Channel16 : Subsystem
  route2Channel17 : Subsystem
  route2Channel18 : Subsystem
  route2Channel2 : Subsystem
  route2Channel3 : Subsystem
  route2Channel4 : Subsystem
  route2Channel5 : Subsystem
  route2Channel6 : Subsystem
  route2Channel7 : Subsystem
  route2Channel8 : Subsystem
  route2Channel9 : Subsystem
  route2recirculate : Subsystem
  toChannel : NServer  NumberOfServers=15  ServiceTime=6
  toChannel{1..18} (18 alike) : NServer  NumberOfServers=2  ServiceTime=0.8
  toMainConveyor : NServer  ServiceTime=2
  toRecirculate : NServer  NumberOfServers=3
  toVerify : NServer  NumberOfServers=12  ServiceTime=5  StatNumberInBlock=on
      settings: OutputPortMap=o1
  toVerify{1..17} (17 alike) : NServer  NumberOfServers=2  ServiceTime=0.8
  verifyWorkstation : Subsystem
  toMHS : PMIOPort  Port=1  Side=Left
  fromMHS : PMIOPort  Port=2  Side=Left
  WIP : Outport
  wires:
  fillChannel1/1(serverAvailable) -> route2Channel1/1(serverAvailable)
  INFlowCount/1 -> Add1/1
  OUTFlowCount/1 -> Add1/2
  Add1/1 -> WIP/1
  fillChannel2/1(serverAvailable) -> route2Channel2/1(serverAvailable)
  fillChannel3/1(serverAvailable) -> route2Channel3/1(serverAvailable)
  fillChannel4/1(serverAvailable) -> route2Channel4/1(serverAvailable)
  fillChannel5/1(serverAvailable) -> route2Channel5/1(serverAvailable)
  fillChannel6/1(serverAvailable) -> route2Channel6/1(serverAvailable)
  fillChannel7/1(serverAvailable) -> route2Channel7/1(serverAvailable)
  fillChannel8/1(serverAvailable) -> route2Channel8/1(serverAvailable)
  fillChannel9/1(serverAvailable) -> route2Channel9/1(serverAvailable)
  fillChannel10/1(serverAvailable) -> route2Channel10/1(serverAvailable)
  fillChannel11/1(serverAvailable) -> route2Channel11/1(serverAvailable)
  fillChannel12/1(serverAvailable) -> route2Channel12/1(serverAvailable)
  fillChannel13/1(serverAvailable) -> route2Channel13/1(serverAvailable)
  fillChannel14/1(serverAvailable) -> route2Channel14/1(serverAvailable)
  fillChannel15/1(serverAvailable) -> route2Channel15/1(serverAvailable)
  fillChannel16/1(serverAvailable) -> route2Channel16/1(serverAvailable)
  fillChannel17/1(serverAvailable) -> route2Channel17/1(serverAvailable)
  fillChannel18/1(serverAvailable) -> route2Channel18/1(serverAvailable)
  toVerify/1 -> route2recirculate/1(verifyQueueLength)
  verifyWorkstation/1(queueLength) -> ?
  connections:
  fillChannel1/LConn1 -- route2Channel1/RConn1
  toChannel1/RConn1 -- route2Channel1/LConn1
  combineRecirculate/RConn1 -- toChannel1/LConn1
  route2recirculate/RConn1 -- combineRecirculate/LConn1
  OUTFlowCount/RConn1 -- toMHS/RConn1
  fromMHS/RConn1 -- INFlowCount/LConn1
  fillChannel1/RConn1 -- fromChannel1/LConn2
  toRecirculate/LConn1 -- fromChannel1/RConn1
  route2recirculate/LConn1 -- toRecirculate/RConn1
  route2Channel2/RConn1 -- fillChannel2/LConn1
  fillChannel2/RConn1 -- fromChannel2/LConn2
  route2Channel2/LConn1 -- toChannel2/RConn1
  toVerify1/LConn1 -- fromChannel2/RConn1
  route2Channel3/RConn1 -- fillChannel3/LConn1
  fillChannel3/RConn1 -- fromChannel3/LConn2
  route2Channel3/LConn1 -- toChannel3/RConn1
  toVerify2/LConn1 -- fromChannel3/RConn1
  route2Channel4/RConn1 -- fillChannel4/LConn1
  fillChannel4/RConn1 -- fromChannel4/LConn2
  route2Channel4/LConn1 -- toChannel4/RConn1
  toVerify3/LConn1 -- fromChannel4/RConn1
  route2Channel5/RConn1 -- fillChannel5/LConn1
  fillChannel5/RConn1 -- fromChannel5/LConn2
  route2Channel5/LConn1 -- toChannel5/RConn1
  toVerify4/LConn1 -- fromChannel5/RConn1
  route2Channel6/RConn1 -- fillChannel6/LConn1
  fillChannel6/RConn1 -- fromChannel6/LConn2
  route2Channel6/LConn1 -- toChannel6/RConn1
  toVerify5/LConn1 -- fromChannel6/RConn1
  route2Channel7/RConn1 -- fillChannel7/LConn1
  fillChannel7/RConn1 -- fromChannel7/LConn2
  route2Channel7/LConn1 -- toChannel7/RConn1
  toVerify6/LConn1 -- fromChannel7/RConn1
  route2Channel8/RConn1 -- fillChannel8/LConn1
  fillChannel8/RConn1 -- fromChannel8/LConn2
  route2Channel8/LConn1 -- toChannel8/RConn1
  toVerify7/LConn1 -- fromChannel8/RConn1
  route2Channel9/RConn1 -- fillChannel9/LConn1
  fillChannel9/RConn1 -- fromChannel9/LConn2
  route2Channel9/LConn1 -- toChannel9/RConn1
  toVerify8/LConn1 -- fromChannel9/RConn1
  fromChannel1/LConn1 -- toVerify1/RConn1
  route2Channel1/RConn2 -- toChannel2/LConn1
  route2Channel2/RConn2 -- toChannel3/LConn1
  fromChannel2/LConn1 -- toVerify2/RConn1
  fromChannel3/LConn1 -- toVerify3/RConn1
  route2Channel3/RConn2 -- toChannel4/LConn1
  fromChannel4/LConn1 -- toVerify4/RConn1
  route2Channel4/RConn2 -- toChannel5/LConn1
  fromChannel5/LConn1 -- toVerify5/RConn1
  route2Channel5/RConn2 -- toChannel6/LConn1
  fromChannel6/LConn1 -- toVerify6/RConn1
  route2Channel6/RConn2 -- toChannel7/LConn1
  fromChannel7/LConn1 -- toVerify7/RConn1
  route2Channel7/RConn2 -- toChannel8/LConn1
  fromChannel8/LConn1 -- toVerify8/RConn1
  route2Channel8/RConn2 -- toChannel9/LConn1
  route2Channel10/RConn2 -- toChannel11/LConn1
  route2Channel12/LConn1 -- toChannel12/RConn1
  route2Channel18/RConn1 -- fillChannel18/LConn1
  fromChannel17/LConn1 -- toVerify17/RConn1
  route2Channel13/RConn2 -- toChannel14/LConn1
  toVerify11/LConn1 -- fromChannel12/RConn1
  fillChannel10/RConn1 -- fromChannel10/LConn2
  fillChannel16/RConn1 -- fromChannel16/LConn2
  toVerify15/LConn1 -- fromChannel16/RConn1
  fromChannel14/LConn1 -- toVerify14/RConn1
  fillChannel15/RConn1 -- fromChannel15/LConn2
  toVerify14/LConn1 -- fromChannel15/RConn1
  route2Channel17/RConn2 -- toChannel18/LConn1
  fromChannel10/LConn1 -- toVerify10/RConn1
  toVerify17/LConn1 -- fromChannel18/RConn1
  route2Channel15/RConn2 -- toChannel16/LConn1
  route2Channel16/LConn1 -- toChannel16/RConn1
  route2Channel11/RConn2 -- toChannel12/LConn1
  toVerify9/LConn1 -- fromChannel10/RConn1
  route2Channel16/RConn2 -- toChannel17/LConn1
  fromChannel15/LConn1 -- toVerify15/RConn1
  toVerify12/LConn1 -- fromChannel13/RConn1
  route2Channel16/RConn1 -- fillChannel16/LConn1
  fromChannel13/LConn1 -- toVerify13/RConn1
  route2Channel15/RConn1 -- fillChannel15/LConn1
  fromChannel16/LConn1 -- toVerify16/RConn1
  route2Channel12/RConn1 -- fillChannel12/LConn1
  fillChannel18/RConn1 -- fromChannel18/LConn2
  route2Channel15/LConn1 -- toChannel15/RConn1
  route2Channel12/RConn2 -- toChannel13/LConn1
  route2Channel18/LConn1 -- toChannel18/RConn1
  fillChannel12/RConn1 -- fromChannel12/LConn2
  route2Channel14/RConn2 -- toChannel15/LConn1
  fromChannel11/LConn1 -- toVerify11/RConn1
  fromChannel12/LConn1 -- toVerify12/RConn1
  route2Channel13/LConn1 -- toChannel13/RConn1
  route2Channel10/LConn1 -- toChannel10/RConn1
  toVerify13/LConn1 -- fromChannel14/RConn1
  route2Channel17/RConn1 -- fillChannel17/LConn1
  fillChannel14/RConn1 -- fromChannel14/LConn2
  fillChannel11/RConn1 -- fromChannel11/LConn2
  route2Channel10/RConn1 -- fillChannel10/LConn1
  route2Channel11/LConn1 -- toChannel11/RConn1
  fillChannel17/RConn1 -- fromChannel17/LConn2
  route2Channel17/LConn1 -- toChannel17/RConn1
  route2Channel14/LConn1 -- toChannel14/RConn1
  toVerify16/LConn1 -- fromChannel17/RConn1
  route2Channel13/RConn1 -- fillChannel13/LConn1
  fillChannel13/RConn1 -- fromChannel13/LConn2
  route2Channel14/RConn1 -- fillChannel14/LConn1
  route2Channel11/RConn1 -- fillChannel11/LConn1
  toVerify10/LConn1 -- fromChannel11/RConn1
  fromChannel9/LConn1 -- toVerify9/RConn1
  route2Channel9/RConn2 -- toChannel10/LConn1
  route2Channel18/RConn2 -- fromChannel18/LConn1
  toChannel/RConn1 -- combineRecirculate/LConn2
  INFlowCount/RConn1 -- toChannel/LConn1
  toVerify/RConn1 -- verifyWorkstation/RConn1
  toVerify/LConn1 -- route2recirculate/RConn2
  toMainConveyor/LConn1 -- verifyWorkstation/LConn1
  toMainConveyor/RConn1 -- OUTFlowCount/LConn1
